simulink model "m_Blue_Lady_mdl__R2021b"  (R2021b)
settings: Solver=ode45  StartTime=0.0  StopTime=400  RelTol=1e-3  EnableMultiTasking=on
settings Model: Creator=ToMi  LastModifiedBy=ToMi
settings SolverCC: AlgebraicLoopSolver=TrustRegion
settings DataIOCC: LimitDataPoints=on  SaveFormat=Array  SignalLoggingSaveFormat=ModelDataLogs  ReturnWorkspaceOutputs=off
settings OptimizationCC: InitFltsAndDblsToZero=on  LifeSpan=inf
settings DebuggingCC: SaveWithParameterizedLinksMsg=none  UnderspecifiedInitializationDetection=Classic  MergeDetectMultiDrivingBlocksExec=none  SignalResolutionControl=TryResolveAllWithWarning  SolverPrmCheckMsg=warning  MultiTaskDSMMsg=warning  MultiTaskCondExecSysMsg=none  FcnCallInpInsideContextMsg=warning  SFUnexpectedBacktrackingDiag=warning  SFNoUnconditionalDefaultTransitionDiag=warning  SFExecutionAtInitializationDiag=none  SFMachineParentedDataDiag=warning  ArithmeticOperatorsInVariantConditions=warning
settings HardwareCC: ProdBitPerPointer=32  ProdBitPerSizeT=32  ProdBitPerPtrDiffT=32  ProdLargestAtomicFloat=None  ProdIntDivRoundTo=Undefined  ProdEndianess=Unspecified  ProdWordSize=32  ProdHWDeviceType=32-bit Generic
settings ModelReferenceCC: PropagateSignalLabelsOutOfModel=off
settings CodeAppCC: StateflowObjectComments=on
settings GRTTargetCC: TargetFcnLib=ansi_tfl_tmw.mat  TargetLangStandard=C89/C90 (ANSI)  CombineOutputUpdateFcns=off  GRTInterface=on
settings ConfigComp: CovMetricSettings=dw  CovSaveCumulativeToWorkspaceVar=on  CovSaveSingleToWorkspaceVar=on

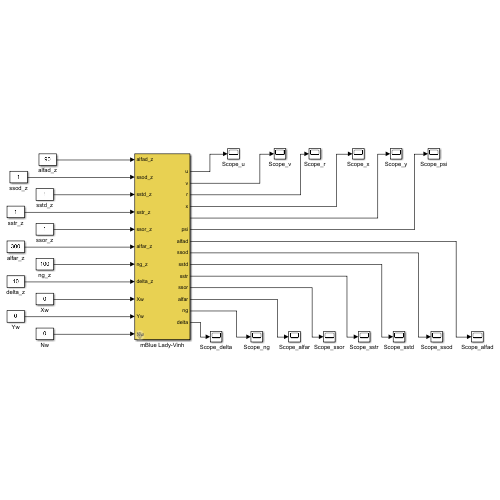
[thumbnail: Simulink's stored preview of the top-level diagram]
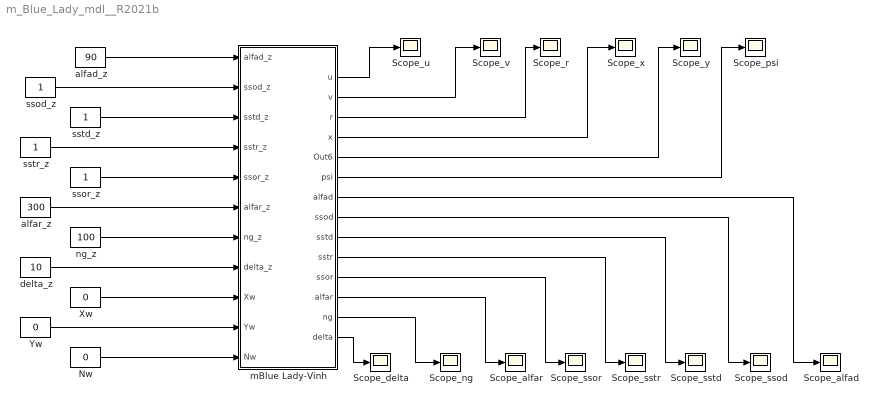
== system m_Blue_Lady_mdl__R2021b ==
  Nw : Constant  Value=0
  Scope_alfad : Scope
  Scope_alfar : Scope
  Scope_delta : Scope
  Scope_ng : Scope
  Scope_psi : Scope
  Scope_r : Scope
  Scope_ssod : Scope
  Scope_ssor : Scope
  Scope_sstd : Scope
  Scope_sstr : Scope
  Scope_u : Scope
  Scope_v : Scope
  Scope_x : Scope
  Scope_y : Scope
  Xw : Constant  Value=0
  Yw : Constant  Value=0
  alfad_z : Constant  Value=90
  alfar_z : Constant  Value=300
  delta_z : Constant  Value=10
  mBlue Lady-Vinh : Subsystem  mask{U_INI=0, V_INI=0, R_INI=0, X_INI=0, Y_INI=0, KURS_INI=0, S_ZAL=Full}
      mask prompts: U_INI "u0 ="; V_INI "v0 ="; R_INI "r0 ="; X_INI "Xo ="; Y_INI "Yo ="; KURS_INI "Kurs0 ="; S_ZAL "Stan zaladowania"
      mask TypeOptions S_ZAL: Balast | Full
  ng_z : Constant  Value=100
  ssod_z : Constant
  ssor_z : Constant
  sstd_z : Constant
  sstr_z : Constant
  wires:
  delta_z/1 -> mBlue Lady-Vinh/8(delta_z)
  alfad_z/1 -> mBlue Lady-Vinh/1(alfad_z)
  ssod_z/1 -> mBlue Lady-Vinh/2(ssod_z)
  sstd_z/1 -> mBlue Lady-Vinh/3(sstd_z)
  sstr_z/1 -> mBlue Lady-Vinh/4(sstr_z)
  ssor_z/1 -> mBlue Lady-Vinh/5(ssor_z)
  alfar_z/1 -> mBlue Lady-Vinh/6(alfar_z)
  ng_z/1 -> mBlue Lady-Vinh/7(ng_z)
  Xw/1 -> mBlue Lady-Vinh/9(Xw)
  Yw/1 -> mBlue Lady-Vinh/10(Yw)
  mBlue Lady-Vinh/1(u) -> Scope_u/1
  mBlue Lady-Vinh/2(v) -> Scope_v/1
  mBlue Lady-Vinh/3(r) -> Scope_r/1
  mBlue Lady-Vinh/4(x) -> Scope_x/1
  mBlue Lady-Vinh/5(Out6) -> Scope_y/1
  mBlue Lady-Vinh/6(psi) -> Scope_psi/1
  mBlue Lady-Vinh/7(alfad) -> Scope_alfad/1
  mBlue Lady-Vinh/8(ssod) -> Scope_ssod/1
  mBlue Lady-Vinh/9(sstd) -> Scope_sstd/1
  mBlue Lady-Vinh/10(sstr) -> Scope_sstr/1
  mBlue Lady-Vinh/11(ssor) -> Scope_ssor/1
  mBlue Lady-Vinh/12(alfar) -> Scope_alfar/1
  mBlue Lady-Vinh/13(ng) -> Scope_ng/1
  mBlue Lady-Vinh/14(delta) -> Scope_delta/1
  Nw/1 -> mBlue Lady-Vinh/11(Nw)

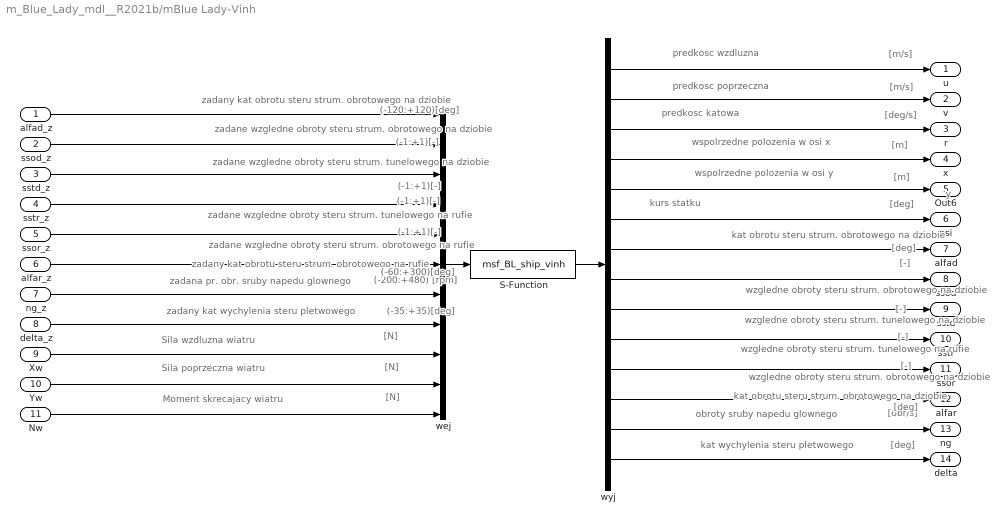
== system m_Blue_Lady_mdl__R2021b/mBlue Lady-Vinh ==
  note: y
  note: predkosc wzdluzna
  note: predkosc poprzeczna
  note: predkosc katowa
  note: kurs statku
  note: wspolrzedne polozenia w osi x
  note: wspolrzedne polozenia w osi y
  note: obroty sruby napedu glownego
  note: kat wychylenia steru pletwowego
  note: wzgledne obroty steru strum. tunelowego na dziobie
  note: wzgledne obroty steru strum. tunelowego na rufie
  note: wzgledne obroty steru strum. obrotowego na dziobie
  note: kat obrotu steru strum. obrotowego na dziobie
  note: wzgledne obroty steru strum. obrotowego na dziobie
  note: kat obrotu steru strum. obrotowego na dziobie
  note: [m/s]
  note: [m/s]
  note: [deg/s]
  note: [deg]
  note: [m]
  note: [m]
  note: [obr/s]
  note: [deg]
  note: [-]
  note: [-]
  note: [-]
  note: [deg]
  note: [-]
  note: [deg]
  note: zadana pr. obr. sruby napedu glownego
  note: (-200:+480) [rpm]
  note: zadany kat wychylenia steru pletwowego
  note: (-35:+35)[deg]
  note: zadane wzgledne obroty steru strum. tunelowego na dziobie
  note: (-1:+1)[-]
  note: zadane wzgledne obroty steru strum. tunelowego na rufie
  note: zadane wzgledne obroty steru strum. obrotowego na dziobie
  note: zadany kat obrotu steru strum. obrotowego na dziobie
  note: zadane wzgledne obroty steru strum. obrotowego na rufie
  note: zadany kat obrotu steru strum. obrotowego na rufie
  note: Sila wzdluzna wiatru
  note: Sila poprzeczna wiatru
  note: (-1:+1)[-]
  note: (-1:+1)[-]
  note: (-1:+1)[-]
  note: (-120:+120)[deg]
  note: (-60:+300)[deg]
  note: [N]
  note: [N]
  note: Moment skrecajacy wiatru
  note: [N]
  alfad_z : Inport
  ssod_z : Inport  Port=2
  sstd_z : Inport  Port=3
  sstr_z : Inport  Port=4
  ssor_z : Inport  Port=5
  alfar_z : Inport  Port=6
  ng_z : Inport  Port=7
  delta_z : Inport  Port=8
  Xw : Inport  Port=9
  Yw : Inport  Port=10
  Nw : Inport  Port=11
  S-Function : S-Function  FunctionName=msf_BL_ship_vinh  Parameters=U_INI, V_INI, R_INI, X_INI, Y_INI, KURS_INI, S_ZAL  SFunctionDeploymentMode=off  EnableBusSupport=off
  wej : Mux  Inputs=11
  wyj : Demux  Outputs=14
      settings: DisplayOption=none
  u : Outport  InitialOutput=0
  v : Outport  Port=2  InitialOutput=0
  r : Outport  Port=3  InitialOutput=0
  x : Outport  Port=4  InitialOutput=0
  Out6 : Outport  Port=5  InitialOutput=0
  psi : Outport  Port=6  InitialOutput=0
  alfad : Outport  Port=7  InitialOutput=0
  ssod : Outport  Port=8  InitialOutput=0
  sstd : Outport  Port=9  InitialOutput=0
  sstr : Outport  Port=10  InitialOutput=0
  ssor : Outport  Port=11  InitialOutput=0
  alfar : Outport  Port=12  InitialOutput=0
  ng : Outport  Port=13  InitialOutput=0
  delta : Outport  Port=14  InitialOutput=0
  wires:
  wej/1 -> S-Function/1
  S-Function/1 -> wyj/1
  alfad_z/1 -> wej/1
  ssod_z/1 -> wej/2
  sstd_z/1 -> wej/3
  sstr_z/1 -> wej/4
  ssor_z/1 -> wej/5
  alfar_z/1 -> wej/6
  ng_z/1 -> wej/7
  delta_z/1 -> wej/8
  Xw/1 -> wej/9
  Yw/1 -> wej/10
  wyj/1 -> u/1
  wyj/2 -> v/1
  wyj/3 -> r/1
  wyj/4 -> x/1
  wyj/5 -> Out6/1
  wyj/6 -> psi/1
  wyj/7 -> alfad/1
  wyj/8 -> ssod/1
  wyj/9 -> sstd/1
  wyj/10 -> sstr/1
  wyj/11 -> ssor/1
  wyj/12 -> alfar/1
  wyj/13 -> ng/1
  wyj/14 -> delta/1
  Nw/1 -> wej/11
